simulink model "IEEE34bus_2subsystem"  (R2022b)
settings: Solver=ode4  StartTime=0.0  StopTime=inf  FixedStep=Ts  MaxStep=1e-4  RelTol=1e-4
InitFcn:
  | a=1; % Loading Factor
  | Ts=50e-6;
  | % phase to sequence conversion of RXB matrices
  | c=1*exp(sqrt(-1)*(120*pi/180));
  | T=[1 1 1;1 c*c c;1 c c*c];
  | Tinv=1/3*[1 1 1;1 c c*c;1 c*c c];
  | 
  | % Simulation data for the IEEE 34 Node Test Feeder model
  | mi2km = 1.60934;%  miles to km conversion
  | ft2km = 0.0003048; % feet to km conversion
  | ms2F = 1*1e-6/(2*pi*60);% microsiemens to Farads conversion
  | 
  | %% Configuration 300 - series reactance - ohm/mile
  | R_300 = [1.3368 0.2101 0.2130;0.2101 1.3238 0.2066;0.2130 0.2066 1.3294];
  | X_300 = [1.3343 0.5779 0.5015;0.5779 1.3569 0.4591;0.5015 0.4591 1.3471];
  | % charging susceptance - microsiemens/mile
  | B_300 = [5.3350 -1.5313 -0.9943;-1.5313 5.0979 -0.6212;-0.9943 -0.6212 4.8880];
  | 
  | R_300 = R_300/mi2km;
  | Rseq=Tinv*R_300*T;
  | R1_300=Rseq(2,2);R0_300=Rseq(1,1);
  | 
  | L_300 = (X_300/(2*pi*60))/mi2km;
  | Lseq=Tinv*L_300*T;
  | L1_300=Lseq(2,2);L0_300=Lseq(1,1);
  | 
  | C_300 =(B_300*ms2F)/mi2km;
  | Cseq=Tinv*C_300*T;
  | C1_300=Cseq(2,2);C0_300=Cseq(1,1);
  | 
  | %% Configuration 301 - series reactance - ohm/mile
  | R_301 = [1.9300 0.2327 0.2359;0.2327 1.9157 0.2288;0.2359 0.2288 1.9219];
  | X_301 = [1.4115 0.6442 0.5691;0.6442 1.4281 0.5238;0.5691 0.5238 1.4209];
  | % charging susceptance - microsiemens/mile
  | B_301 = [5.1207 -1.4364 -0.9402;-1.4364 4.9055 -0.5951;-0.9402 -0.5951 4.7154];
  | 
  | R_301 = R_301/mi2km;
  | Rseq=Tinv*R_301*T;
  | R1_301=Rseq(2,2);R0_301=Rseq(1,1);
  | 
  | L_301 = (X_301/(2*pi*60))/mi2km;
  | Lseq=Tinv*L_301*T;
  | L1_301=Lseq(2,2);L0_301=Lseq(1,1);
  | 
  | C_301 =(B_301*ms2F)/mi2km;
  | Cseq=Tinv*C_301*T;
  | C1_301=Cseq(2,2);C0_301=Cseq(1,1);
  | 
  | %% Configuration 302 - series reactance - ohm/mile
  | R_302 = [2.7995 0 0;0 0 0;0 0 0];
  | X_302 = [1.4855 0 0;0 0 0;0 0 0];
  | % charging susceptance - microsiemens/mile
  | B_302 = [4.2251 0 0;0 0 0;0 0 0];
  | 
  | R_302 = R_302/mi2km;
  | Rseq=Tinv*R_302*T;
  | R1_302=Rseq(2,2);R0_302=Rseq(1,1);
  | 
  | L_302 = (X_302/(2*pi*60))/mi2km;
  | Lseq=Tinv*L_302*T;
  | ... (+41 lines)
undefined symbols (not defined in the file): find_system, I, Left, MOV_segment19, MOV_segment9, powergui, Right, type, V, X, xn_g1
libraries: spsSeriesRLCBranchLib x75, spsGroundLib x70, spsThreePhaseVIMeasurementLib x37, spsVoltageMeasurementLib x36, spsThreePhaseSeriesRLCLoadLib x32, spsThreePhasePISectionLineLib x24, spsDCVoltageSourceLib x24, ssn_lib x16, spsSeriesRLCLoadLib x14, spsACCurrentSourceLib x12, spsOnDelayLib x12, spsPiSectionLineLib x8
(part 6 of 8)

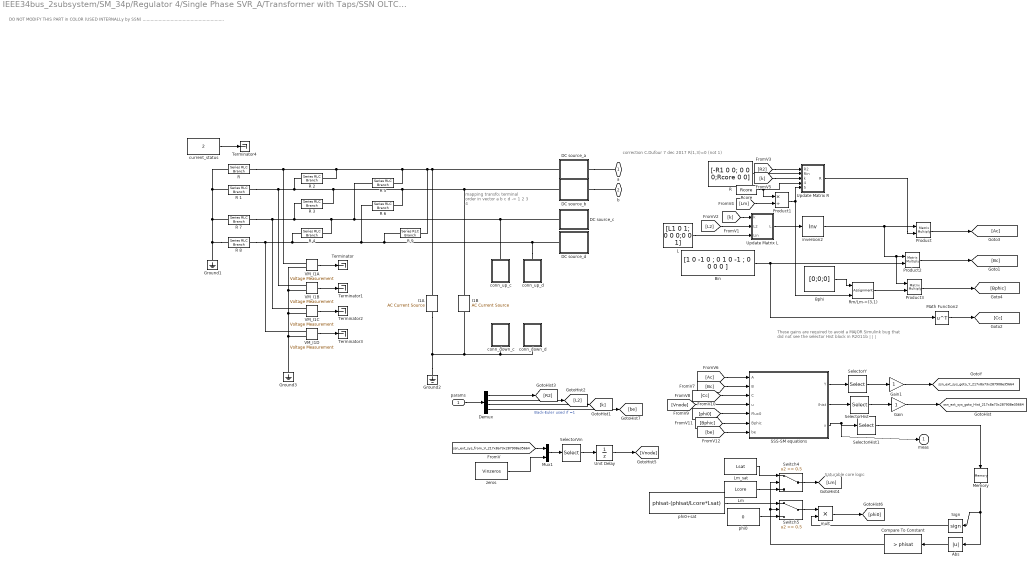
== system IEEE34bus_2subsystem/SM_34p/Regulator 4/Single Phase SVR_A/Transformer with Taps/SSN OLTC xfo v2 ==
  note: correction C.Dufour 7 dec 2017 R(1,3)=0 (not 1)
  note: These gains are required to avoid a MAJOR Simulink bug
      | that did not see the selector Hist block in R2011b
      | |
      | |
      | |
  note: Saturable core logic
  note: DO NOT MODIFY THIS PART in COLOR (USED INTERNALLy by SSN) .............................................................
  note: mapping transfo:
      | terminal    order in vector
      | a b c d -> 1 2 3 4
  params : Inport
  Abs : Abs  SaturateOnIntegerOverflow=off
  Bin : Constant  Value="[1 0 -1  0 ; 0 1 0 -1 ; 0 0 0 0 ]"
  Bphi : Constant  Value=[0;0;0]  VectorParams1D=off
  Compare To Constant : simulink/Logic and Bit Operations/Compare To Constant  relop=>  const=phisat  OutDataTypeStr=uint8
  DC source_a : Subsystem  mask(SSN nodal point interface: DC-source){}
  DC source_b : Subsystem  mask(SSN nodal point interface: DC-source){}
  DC source_c : Subsystem  mask(SSN nodal point interface: DC-source){}
  DC source_d : Subsystem  mask(SSN nodal point interface: DC-source){}
  Demux : Demux
  Gain : Gain
  Gain1 : Gain
  Ground1 : spsGroundLib/Ground  LConnTagsString=a
  Ground2 : spsGroundLib/Ground  LConnTagsString=a
  Ground3 : spsGroundLib/Ground  LConnTagsString=a
  I1A : spsACCurrentSourceLib/AC Current Source  Amplitude=0  Phase=0  Frequency=1928.3746  SampleTime=0  Measurements=None
      settings: LibrarySourceBlock=sps_lib/Sources/AC Current Source
  I1B : spsACCurrentSourceLib/AC Current Source  Amplitude=0  Phase=0  Frequency=1928.3746  SampleTime=0  Measurements=None
      settings: LibrarySourceBlock=sps_lib/Sources/AC Current Source
  L : Constant  Value=[L1 0 1; 0 0 0;0 0 1]
  Lm : Constant  Value=Lcore
  Lm_sat : Constant  Value=Lsat
  Math Function2 : Math  Operator=transpose  SignedPower=on
  Memory : Memory
  Mux1 : Mux  Inputs=2
  Product : Product  Multiplication=Matrix(*)  RndMeth=Zero
  Product1 : Product  Inputs=*/  RndMeth=Zero
  Product2 : Product  Multiplication=Matrix(*)  RndMeth=Zero
  Product3 : Product  Multiplication=Matrix(*)  RndMeth=Zero
  R : Constant  Value=[-R1 0 0; 0 0 0;Rcore 0 0]
  R {,1..9} (10 alike) : spsSeriesRLCBranchLib/Series RLC Branch  LConnTagsString=__new0  RConnTagsString=__new0  BranchType=R  Resistance=1.23456789  Inductance=.5  SetiL0=off  InitialCurrent=0  Capacitance=1.0  Setx0=off  InitialVoltage=0  Measurements=None
  Rcore : Constant  Value=Rcore
  "Rm/Lm->(3,1) " : Assignment  NumberOfDimensions=2  IndexOptions=Index vector (dialog),Index vector (dialog)  Indices=3,1  OutputSizes=1,1
  SSS-SM equations : Subsystem
  SelectorHist : Selector  InputPortWidth=4  IndexOptions=Index vector (dialog)  Indices=hist_sel  OutputSizes=1
  SelectorHist1 : Selector  InputPortWidth=3  IndexOptions=Index vector (dialog)  Indices=3  OutputSizes=1
  SelectorVin : Selector  InputPortWidth=5  IndexOptions=Index vector (dialog)  Indices=vin_sel  OutputSizes=1
  SelectorY : Selector  NumberOfDimensions=2  InputPortWidth=4  IndexOptions=Index vector (dialog),Index vector (dialog)  Indices=hist_sel,hist_sel  OutputSizes=1,1
  Sign : Signum
  Switch4 : Switch  Threshold=0.5  SaturateOnIntegerOverflow=off  InputSameDT=off
  Switch5 : Switch  Threshold=0.5  SaturateOnIntegerOverflow=off  InputSameDT=off
  Terminator{,1..4} (5 alike) : Terminator
  Unit Delay : UnitDelay  SampleTime=Ts  HasFrameUpgradeWarning=on
  Update Matrix L : Subsystem
  Update Matrix R : Subsystem
  VM_I1A : spsVoltageMeasurementLib/Voltage Measurement  PhasorSimulation=off  OutputType=Complex  PSBequivalent=0
  VM_I1B : spsVoltageMeasurementLib/Voltage Measurement  PhasorSimulation=off  OutputType=Complex  PSBequivalent=0
  VM_I1C : spsVoltageMeasurementLib/Voltage Measurement  PhasorSimulation=off  OutputType=Complex  PSBequivalent=0
  VM_I1D : spsVoltageMeasurementLib/Voltage Measurement  PhasorSimulation=off  OutputType=Complex  PSBequivalent=0
  conn_down_c : Subsystem
  conn_down_d : Subsystem
  conn_up_c : Subsystem
  conn_up_d : Subsystem
  current_status : Constant  Value=2
  inversion2 : Product  Inputs=/  Multiplication=Matrix(*)  RndMeth=Zero
  mult : Product
  phi0 : Constant  Value=0
  phi0+sat : Constant  Value=phisat-(phisat/Lcore*Lsat)
  zeros : Constant  Value=Vinzeros
  a : PMIOPort  Side=Left
  b : PMIOPort  Port=2  Side=Right
  meas : Outport  InitialOutput=0  VectorParamsAs1DForOutWhenUnconnected=off
  tag scope: ssn_ext_sys_goto_Hist_217x8a73x287908e35664=global, ssn_ext_sys_goto_Y_217x8a73x287908e35664=global
  wires:
  Gain1/1 -> [ssn_ext_sys_goto_Y_217x8a73x287908e35664]
  Gain/1 -> [ssn_ext_sys_goto_Hist_217x8a73x287908e35664]
  Sign/1 -> mult/2
  mult/1 -> [phi0]
  Switch5/1 -> mult/1
  Unit Delay/1 -> [Vnode]
  params/1 -> Demux/1
  Demux/1 -> [R2]
  Demux/2 -> [L2]
  Demux/3 -> [k]
  Abs/1 -> Compare To Constant/1
  Lm_sat/1 -> Switch4/1
  Lm/1 -> Switch4/3
  Memory/1 -> Abs/1, Sign/1
  phi0/1 -> Switch5/3
  phi0+sat/1 -> Switch5/1
  Switch4/1 -> [Lm]
  Compare To Constant/1 -> Switch4/2, Switch5/2
  [ssn_ext_sys_from_V_217x8a73x287908e35664] -> Mux1/1
  zeros/1 -> Mux1/2
  SelectorVin/1 -> Unit Delay/1
  Mux1/1 -> SelectorVin/1
  current_status/1 -> Terminator4/1
  VM_I1D/1 -> Terminator3/1
  VM_I1C/1 -> Terminator2/1
  VM_I1B/1 -> Terminator1/1
  VM_I1A/1 -> Terminator/1
  L/1 -> Update Matrix L/3(Lin)
  [k] -> Update Matrix L/1(k)
  [L2] -> Update Matrix L/2(L2)
  Update Matrix L/1(L) -> inversion2/1
  R/1 -> Update Matrix R/2(Rin)
  [R2] -> Update Matrix R/1(R2)
  [k] -> Update Matrix R/3(k)
  Rcore/1 -> Update Matrix R/4(Rcore), Product1/1
  inversion2/1 -> Product2/1, Product3/1, Product/1
  [Lm] -> Product1/2
  Product1/1 -> Update Matrix R/5(Rcore/Lcore), "Rm/Lm->(3,1) "/2
  Bin/1 -> Math Function2/1, Product2/2
  Math Function2/1 -> [Cc]
  [Ac] -> SSS-SM equations/1(A)
  [Bc] -> SSS-SM equations/2(B)
  [Cc] -> SSS-SM equations/3(C)
  [Vnode] -> SSS-SM equations/4(u)
  [phi0] -> SSS-SM equations/5(Flux0)
  Bphi/1 -> "Rm/Lm->(3,1) "/1
  [Bphic] -> SSS-SM equations/6(Bphic)
  Product2/1 -> [Bc]
  "Rm/Lm->(3,1) "/1 -> Product3/2
  Update Matrix R/1(R) -> Product/2
  Product/1 -> [Ac]
  Product3/1 -> [Bphic]
  SSS-SM equations/3(x) -> SelectorHist1/1, meas/1
  SelectorHist1/1 -> Memory/1
  [be] -> SSS-SM equations/7(be)
  Demux/4 -> [be]  "Back-Euler used if =1"
  SSS-SM equations/2(Ihist) -> SelectorHist/1
  SSS-SM equations/1(Y) -> SelectorY/1
  SelectorY/1 -> Gain1/1
  SelectorHist/1 -> Gain/1
  connections:
  R 5/RConn1 -- VM_I1A/LConn1 -- "R "/RConn1 -- R 2/RConn1 -- I1A/RConn1 -- DC source_a/LConn1 -- R 9/RConn1
  R 3/RConn1 -- VM_I1B/LConn1 -- R 1/RConn1 -- R 2/LConn1 -- I1B/RConn1 -- DC source_b/LConn1 -- R 6/RConn1
  R 4/RConn1 -- VM_I1C/LConn1 -- R 7/RConn1 -- R 3/LConn1 -- conn_up_c/LConn1 -- DC source_c/LConn1 -- R 5/LConn1
  conn_up_d/LConn1 -- DC source_d/LConn1 -- R 9/LConn1 -- R 6/LConn1 -- VM_I1D/LConn1 -- R 8/RConn1 -- R 4/LConn1
  Ground3/LConn1 -- VM_I1C/LConn2 -- VM_I1A/LConn2 -- VM_I1B/LConn2 -- VM_I1D/LConn2
  DC source_b/RConn1 -- b/RConn1
  Ground2/LConn1 -- I1A/LConn1 -- I1B/LConn1 -- conn_down_c/RConn1 -- conn_down_d/RConn1
  DC source_a/RConn1 -- a/RConn1
  R 8/LConn1 -- Ground1/LConn1 -- R 7/LConn1 -- R 1/LConn1 -- "R "/LConn1

== system IEEE34bus_2subsystem/SM_34p/Regulator 4/Single Phase SVR_A/Voltage Regulator Control/Tap Changer Control ==
  "Up " : Inport
  "Down " : Inport  Port=2
  Constant : Constant  Value=-1
  Constant1 : Constant
  Determine tap position : Subsystem
  Edge Detector : Subsystem  DialogController=POWERSYS.PowerSysDialog  mask(Edge Detector){model=Rising, ic=0}
      mask prompts: model "Edge:"; ic "Input at t = -eps:"
      mask help:
      | This block compares its present input to its previous input.
      |
      | If the input  is a logic signal (TRUE (1) or FALSE (0), the output is a one-step boolean signal TRUE  when  the specified edge (Rising, Falling or Either)  is detected.
      |
      | This block can also be used to detect the slope polarity of a continuous signal. For example, if the specified edge is  "Rising", the output is TRUE as long as the slope of the input signal is positive.
      |
      | The input value at time preceding t=0 is specified by the parameter "Input at t=-eps"
      mask init: same as IEEE34bus_2subsystem/SM_34p/Regulator 3/Single Phase SVR_A/Voltage Regulator Control/Tap Changer Control/Edge Detector
      mask Help: This block is part of a subset of blocks in the Extras library that does not have documentation associated with it, other than the block mask description.
      mask TypeOptions model: Rising | Falling | Either
      mask Display: plot(0,0,100,100, X1,Y1,X2,Y2,X3,Y3,X4,Y4);
  Logical Operator : Logic  Operator=OR  AllPortsSameDT=off
  Logical Operator1 : Logic  AllPortsSameDT=off
  Mechanical Delay : TransportDelay  DelayTime=MecDelay  InitialOutput=InitialPosition  BufferSize=5120
  Memory : Memory  InitialCondition=1  InheritSampleTime=on
  Relational Operator : RelationalOperator  Operator===  OutDataTypeStr=float('double')  InputSameDT=off
  Switch : Switch  Threshold=0.5  InputSameDT=off
  TapNo : Outport  VectorParamsAs1DForOutWhenUnconnected=off
  Ready : Outport  Port=2  VectorParamsAs1DForOutWhenUnconnected=off
  wires:
  Edge Detector/1(Out) -> Logical Operator1/2
  Logical Operator/1 -> Edge Detector/1(In)
  Memory/1 -> Ready/1, Logical Operator1/1
  Relational Operator/1 -> Memory/1
  Determine tap position/1(TapNo) -> Relational Operator/1, Mechanical Delay/1
  Switch/1 -> Determine tap position/1(NewTap)
  Constant1/1 -> Switch/3
  Constant/1 -> Switch/1
  "Down "/1 -> Switch/2, Logical Operator/2
  "Up "/1 -> Logical Operator/1
  Logical Operator1/1 -> Determine tap position/Trigger
  Mechanical Delay/1 -> Relational Operator/2, TapNo/1

== system IEEE34bus_2subsystem/SM_34p/Regulator 4/Single Phase SVR_A/Voltage Regulator Control/Voltage regulator ==
  Vmes (pu) : Inport
  Ready : Inport  Port=2
  RegOn : Inport  Port=3
  Dead Zone : DeadZone  LowerValue=-DeadBand/2  UpperValue=+DeadBand/2
  Discrete Variable Time Delay : spsDiscreteVariableTimeDelayLib/Discrete Variable Time Delay  MaxDelay=3/60+Ts  InitialValue=1  Ts=Ts  DFT=on
      settings: LibrarySourceBlock=|
      | sps_lib/Control/Discrete Variable
      | Time Delay
  Logical Operator : Logic  AllPortsSameDT=off
  Logical Operator1 : Logic  AllPortsSameDT=off
  On Delay : spsOnDelayLib/On Delay  DelayType=On delay  delay=TimeDelay  ic=0  Ts=Ts
  On Delay1 : spsOnDelayLib/On Delay  DelayType=On delay  delay=TimeDelay  ic=0  Ts=Ts
  Relational Operator : RelationalOperator  Operator=>  InputSameDT=off
  Relational Operator1 : RelationalOperator  Operator=<  InputSameDT=off
  Sum : Sum  Inputs=|+-  SaturateOnIntegerOverflow=on
  Switch : Switch  Threshold=1.5  InputSameDT=off
  Vref : Constant  Value=Vref
  Vref1 : Constant  Value=0
  Vref2 : Constant  Value=0
  Vref3 : Constant  Value=0
  Vref4 : Constant  Value=3/60
  Up : Outport  VectorParamsAs1DForOutWhenUnconnected=off
  Down : Outport  Port=2  VectorParamsAs1DForOutWhenUnconnected=off
  wires:
  Vref4/1 -> Discrete Variable Time Delay/2
  Discrete Variable Time Delay/1 -> Logical Operator/2, Logical Operator1/1
  Vref3/1 -> Relational Operator1/2
  On Delay1/1 -> Down/1
  Logical Operator1/1 -> On Delay1/1
  Relational Operator1/1 -> Logical Operator1/2
  On Delay/1 -> Up/1
  Logical Operator/1 -> On Delay/1
  Ready/1 -> Discrete Variable Time Delay/1
  Relational Operator/1 -> Logical Operator/1
  Vref1/1 -> Relational Operator/2
  Dead Zone/1 -> Relational Operator/1, Relational Operator1/1
  Vmes (pu)/1 -> Sum/2
  Vref/1 -> Sum/1
  Sum/1 -> Switch/1
  Switch/1 -> Dead Zone/1
  RegOn/1 -> Switch/2
  Vref2/1 -> Switch/3

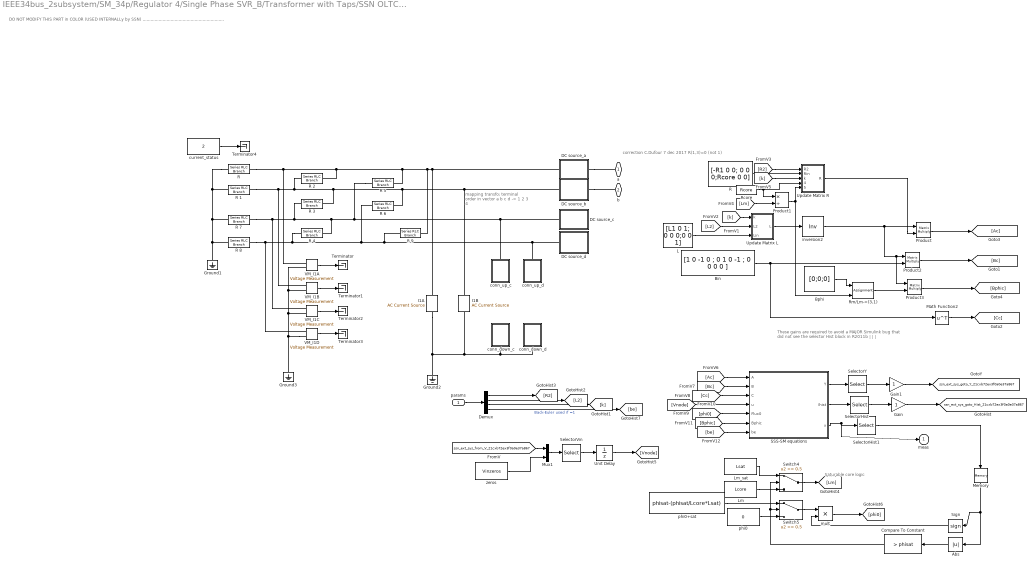
== system IEEE34bus_2subsystem/SM_34p/Regulator 4/Single Phase SVR_B/Transformer with Taps/SSN OLTC xfo v2 ==
  note: mapping transfo:
      | terminal    order in vector
      | a b c d -> 1 2 3 4
  note: DO NOT MODIFY THIS PART in COLOR (USED INTERNALLy by SSN) .............................................................
  note: Saturable core logic
  note: These gains are required to avoid a MAJOR Simulink bug
      | that did not see the selector Hist block in R2011b
      | |
      | |
      | |
  note: correction C.Dufour 7 dec 2017 R(1,3)=0 (not 1)
  params : Inport
  Abs : Abs  SaturateOnIntegerOverflow=off
  Bin : Constant  Value="[1 0 -1  0 ; 0 1 0 -1 ; 0 0 0 0 ]"
  Bphi : Constant  Value=[0;0;0]  VectorParams1D=off
  Compare To Constant : simulink/Logic and Bit Operations/Compare To Constant  relop=>  const=phisat  OutDataTypeStr=uint8
  DC source_a : Subsystem  mask(SSN nodal point interface: DC-source){}
  DC source_b : Subsystem  mask(SSN nodal point interface: DC-source){}
  DC source_c : Subsystem  mask(SSN nodal point interface: DC-source){}
  DC source_d : Subsystem  mask(SSN nodal point interface: DC-source){}
  Demux : Demux
  Gain : Gain
  Gain1 : Gain
  Ground1 : spsGroundLib/Ground  LConnTagsString=a
  Ground2 : spsGroundLib/Ground  LConnTagsString=a
  Ground3 : spsGroundLib/Ground  LConnTagsString=a
  I1A : spsACCurrentSourceLib/AC Current Source  Amplitude=0  Phase=0  Frequency=1928.3746  SampleTime=0  Measurements=None
      settings: LibrarySourceBlock=sps_lib/Sources/AC Current Source
  I1B : spsACCurrentSourceLib/AC Current Source  Amplitude=0  Phase=0  Frequency=1928.3746  SampleTime=0  Measurements=None
      settings: LibrarySourceBlock=sps_lib/Sources/AC Current Source
  L : Constant  Value=[L1 0 1; 0 0 0;0 0 1]
  Lm : Constant  Value=Lcore
  Lm_sat : Constant  Value=Lsat
  Math Function2 : Math  Operator=transpose  SignedPower=on
  Memory : Memory
  Mux1 : Mux  Inputs=2
  Product : Product  Multiplication=Matrix(*)  RndMeth=Zero
  Product1 : Product  Inputs=*/  RndMeth=Zero
  Product2 : Product  Multiplication=Matrix(*)  RndMeth=Zero
  Product3 : Product  Multiplication=Matrix(*)  RndMeth=Zero
  R : Constant  Value=[-R1 0 0; 0 0 0;Rcore 0 0]
  R {,1..9} (10 alike) : spsSeriesRLCBranchLib/Series RLC Branch  LConnTagsString=__new0  RConnTagsString=__new0  BranchType=R  Resistance=1.23456789  Inductance=.5  SetiL0=off  InitialCurrent=0  Capacitance=1.0  Setx0=off  InitialVoltage=0  Measurements=None
  Rcore : Constant  Value=Rcore
  "Rm/Lm->(3,1) " : Assignment  NumberOfDimensions=2  IndexOptions=Index vector (dialog),Index vector (dialog)  Indices=3,1  OutputSizes=1,1
  SSS-SM equations : Subsystem
  SelectorHist : Selector  InputPortWidth=4  IndexOptions=Index vector (dialog)  Indices=hist_sel  OutputSizes=1
  SelectorHist1 : Selector  InputPortWidth=3  IndexOptions=Index vector (dialog)  Indices=3  OutputSizes=1
  SelectorVin : Selector  InputPortWidth=5  IndexOptions=Index vector (dialog)  Indices=vin_sel  OutputSizes=1
  SelectorY : Selector  NumberOfDimensions=2  InputPortWidth=4  IndexOptions=Index vector (dialog),Index vector (dialog)  Indices=hist_sel,hist_sel  OutputSizes=1,1
  Sign : Signum
  Switch4 : Switch  Threshold=0.5  SaturateOnIntegerOverflow=off  InputSameDT=off
  Switch5 : Switch  Threshold=0.5  SaturateOnIntegerOverflow=off  InputSameDT=off
  Terminator{,1..4} (5 alike) : Terminator
  Unit Delay : UnitDelay  SampleTime=Ts  HasFrameUpgradeWarning=on
  Update Matrix L : Subsystem
  Update Matrix R : Subsystem
  VM_I1A : spsVoltageMeasurementLib/Voltage Measurement  PhasorSimulation=off  OutputType=Complex  PSBequivalent=0
  VM_I1B : spsVoltageMeasurementLib/Voltage Measurement  PhasorSimulation=off  OutputType=Complex  PSBequivalent=0
  VM_I1C : spsVoltageMeasurementLib/Voltage Measurement  PhasorSimulation=off  OutputType=Complex  PSBequivalent=0
  VM_I1D : spsVoltageMeasurementLib/Voltage Measurement  PhasorSimulation=off  OutputType=Complex  PSBequivalent=0
  conn_down_c : Subsystem
  conn_down_d : Subsystem
  conn_up_c : Subsystem
  conn_up_d : Subsystem
  current_status : Constant  Value=2
  inversion2 : Product  Inputs=/  Multiplication=Matrix(*)  RndMeth=Zero
  mult : Product
  phi0 : Constant  Value=0
  phi0+sat : Constant  Value=phisat-(phisat/Lcore*Lsat)
  zeros : Constant  Value=Vinzeros
  a : PMIOPort  Side=Left
  b : PMIOPort  Port=2  Side=Right
  meas : Outport  InitialOutput=0  VectorParamsAs1DForOutWhenUnconnected=off
  tag scope: ssn_ext_sys_goto_Hist_21cxb72ex3f0a0e37a867=global, ssn_ext_sys_goto_Y_21cxb72ex3f0a0e37a867=global
  wires:
  SelectorHist/1 -> Gain/1
  SelectorY/1 -> Gain1/1
  SSS-SM equations/1(Y) -> SelectorY/1
  SSS-SM equations/2(Ihist) -> SelectorHist/1
  Demux/4 -> [be]  "Back-Euler used if =1"
  [be] -> SSS-SM equations/7(be)
  SelectorHist1/1 -> Memory/1
  SSS-SM equations/3(x) -> meas/1, SelectorHist1/1
  Product3/1 -> [Bphic]
  Product/1 -> [Ac]
  Update Matrix R/1(R) -> Product/2
  "Rm/Lm->(3,1) "/1 -> Product3/2
  Product2/1 -> [Bc]
  [Bphic] -> SSS-SM equations/6(Bphic)
  Bphi/1 -> "Rm/Lm->(3,1) "/1
  [phi0] -> SSS-SM equations/5(Flux0)
  [Vnode] -> SSS-SM equations/4(u)
  [Cc] -> SSS-SM equations/3(C)
  [Bc] -> SSS-SM equations/2(B)
  [Ac] -> SSS-SM equations/1(A)
  Math Function2/1 -> [Cc]
  Bin/1 -> Product2/2, Math Function2/1
  Product1/1 -> "Rm/Lm->(3,1) "/2, Update Matrix R/5(Rcore/Lcore)
  [Lm] -> Product1/2
  inversion2/1 -> Product/1, Product3/1, Product2/1
  Rcore/1 -> Product1/1, Update Matrix R/4(Rcore)
  [k] -> Update Matrix R/3(k)
  [R2] -> Update Matrix R/1(R2)
  R/1 -> Update Matrix R/2(Rin)
  Update Matrix L/1(L) -> inversion2/1
  [L2] -> Update Matrix L/2(L2)
  [k] -> Update Matrix L/1(k)
  L/1 -> Update Matrix L/3(Lin)
  VM_I1A/1 -> Terminator/1
  VM_I1B/1 -> Terminator1/1
  VM_I1C/1 -> Terminator2/1
  VM_I1D/1 -> Terminator3/1
  current_status/1 -> Terminator4/1
  Mux1/1 -> SelectorVin/1
  SelectorVin/1 -> Unit Delay/1
  zeros/1 -> Mux1/2
  [ssn_ext_sys_from_V_21cxb72ex3f0a0e37a867] -> Mux1/1
  Compare To Constant/1 -> Switch5/2, Switch4/2
  Switch4/1 -> [Lm]
  phi0+sat/1 -> Switch5/1
  phi0/1 -> Switch5/3
  Memory/1 -> Sign/1, Abs/1
  Lm/1 -> Switch4/3
  Lm_sat/1 -> Switch4/1
  Abs/1 -> Compare To Constant/1
  Demux/3 -> [k]
  Demux/2 -> [L2]
  Demux/1 -> [R2]
  params/1 -> Demux/1
  Unit Delay/1 -> [Vnode]
  Switch5/1 -> mult/1
  mult/1 -> [phi0]
  Sign/1 -> mult/2
  Gain/1 -> [ssn_ext_sys_goto_Hist_21cxb72ex3f0a0e37a867]
  Gain1/1 -> [ssn_ext_sys_goto_Y_21cxb72ex3f0a0e37a867]
  connections:
  "R "/LConn1 -- R 1/LConn1 -- R 7/LConn1 -- Ground1/LConn1 -- R 8/LConn1
  DC source_a/RConn1 -- a/RConn1
  conn_down_d/RConn1 -- conn_down_c/RConn1 -- I1B/LConn1 -- I1A/LConn1 -- Ground2/LConn1
  DC source_b/RConn1 -- b/RConn1
  VM_I1D/LConn2 -- VM_I1B/LConn2 -- VM_I1A/LConn2 -- VM_I1C/LConn2 -- Ground3/LConn1
  R 4/LConn1 -- R 8/RConn1 -- VM_I1D/LConn1 -- R 6/LConn1 -- R 9/LConn1 -- DC source_d/LConn1 -- conn_up_d/LConn1
  R 5/LConn1 -- DC source_c/LConn1 -- conn_up_c/LConn1 -- R 3/LConn1 -- R 7/RConn1 -- VM_I1C/LConn1 -- R 4/RConn1
  R 6/RConn1 -- DC source_b/LConn1 -- I1B/RConn1 -- R 2/LConn1 -- R 1/RConn1 -- VM_I1B/LConn1 -- R 3/RConn1
  R 9/RConn1 -- DC source_a/LConn1 -- I1A/RConn1 -- R 2/RConn1 -- "R "/RConn1 -- VM_I1A/LConn1 -- R 5/RConn1

== system IEEE34bus_2subsystem/SM_34p/Regulator 4/Single Phase SVR_B/Voltage Regulator Control/Tap Changer Control ==
  "Up " : Inport
  "Down " : Inport  Port=2
  Constant : Constant  Value=-1
  Constant1 : Constant
  Determine tap position : Subsystem
  Edge Detector : Subsystem  DialogController=POWERSYS.PowerSysDialog  mask(Edge Detector){model=Rising, ic=0}
      mask prompts: model "Edge:"; ic "Input at t = -eps:"
      mask help:
      | This block compares its present input to its previous input.
      |
      | If the input  is a logic signal (TRUE (1) or FALSE (0), the output is a one-step boolean signal TRUE  when  the specified edge (Rising, Falling or Either)  is detected.
      |
      | This block can also be used to detect the slope polarity of a continuous signal. For example, if the specified edge is  "Rising", the output is TRUE as long as the slope of the input signal is positive.
      |
      | The input value at time preceding t=0 is specified by the parameter "Input at t=-eps"
      mask init: same as IEEE34bus_2subsystem/SM_34p/Regulator 3/Single Phase SVR_A/Voltage Regulator Control/Tap Changer Control/Edge Detector
      mask Help: This block is part of a subset of blocks in the Extras library that does not have documentation associated with it, other than the block mask description.
      mask TypeOptions model: Rising | Falling | Either
      mask Display: plot(0,0,100,100, X1,Y1,X2,Y2,X3,Y3,X4,Y4);
  Logical Operator : Logic  Operator=OR  AllPortsSameDT=off
  Logical Operator1 : Logic  AllPortsSameDT=off
  Mechanical Delay : TransportDelay  DelayTime=MecDelay  InitialOutput=InitialPosition  BufferSize=5120
  Memory : Memory  InitialCondition=1  InheritSampleTime=on
  Relational Operator : RelationalOperator  Operator===  OutDataTypeStr=float('double')  InputSameDT=off
  Switch : Switch  Threshold=0.5  InputSameDT=off
  TapNo : Outport  VectorParamsAs1DForOutWhenUnconnected=off
  Ready : Outport  Port=2  VectorParamsAs1DForOutWhenUnconnected=off
  wires:
  Mechanical Delay/1 -> TapNo/1, Relational Operator/2
  Logical Operator1/1 -> Determine tap position/Trigger
  "Up "/1 -> Logical Operator/1
  "Down "/1 -> Logical Operator/2, Switch/2
  Constant/1 -> Switch/1
  Constant1/1 -> Switch/3
  Switch/1 -> Determine tap position/1(NewTap)
  Determine tap position/1(TapNo) -> Mechanical Delay/1, Relational Operator/1
  Relational Operator/1 -> Memory/1
  Memory/1 -> Logical Operator1/1, Ready/1
  Logical Operator/1 -> Edge Detector/1(In)
  Edge Detector/1(Out) -> Logical Operator1/2

== system IEEE34bus_2subsystem/SM_34p/Regulator 4/Single Phase SVR_B/Voltage Regulator Control/Voltage regulator ==
  Vmes (pu) : Inport
  Ready : Inport  Port=2
  RegOn : Inport  Port=3
  Dead Zone : DeadZone  LowerValue=-DeadBand/2  UpperValue=+DeadBand/2
  Discrete Variable Time Delay : spsDiscreteVariableTimeDelayLib/Discrete Variable Time Delay  MaxDelay=3/60+Ts  InitialValue=1  Ts=Ts  DFT=on
      settings: LibrarySourceBlock=|
      | sps_lib/Control/Discrete Variable
      | Time Delay
  Logical Operator : Logic  AllPortsSameDT=off
  Logical Operator1 : Logic  AllPortsSameDT=off
  On Delay : spsOnDelayLib/On Delay  DelayType=On delay  delay=TimeDelay  ic=0  Ts=Ts
  On Delay1 : spsOnDelayLib/On Delay  DelayType=On delay  delay=TimeDelay  ic=0  Ts=Ts
  Relational Operator : RelationalOperator  Operator=>  InputSameDT=off
  Relational Operator1 : RelationalOperator  Operator=<  InputSameDT=off
  Sum : Sum  Inputs=|+-  SaturateOnIntegerOverflow=on
  Switch : Switch  Threshold=1.5  InputSameDT=off
  Vref : Constant  Value=Vref
  Vref1 : Constant  Value=0
  Vref2 : Constant  Value=0
  Vref3 : Constant  Value=0
  Vref4 : Constant  Value=3/60
  Up : Outport  VectorParamsAs1DForOutWhenUnconnected=off
  Down : Outport  Port=2  VectorParamsAs1DForOutWhenUnconnected=off
  wires:
  Vref2/1 -> Switch/3
  RegOn/1 -> Switch/2
  Switch/1 -> Dead Zone/1
  Sum/1 -> Switch/1
  Vref/1 -> Sum/1
  Vmes (pu)/1 -> Sum/2
  Dead Zone/1 -> Relational Operator1/1, Relational Operator/1
  Vref1/1 -> Relational Operator/2
  Relational Operator/1 -> Logical Operator/1
  Ready/1 -> Discrete Variable Time Delay/1
  Logical Operator/1 -> On Delay/1
  On Delay/1 -> Up/1
  Relational Operator1/1 -> Logical Operator1/2
  Logical Operator1/1 -> On Delay1/1
  On Delay1/1 -> Down/1
  Vref3/1 -> Relational Operator1/2
  Discrete Variable Time Delay/1 -> Logical Operator1/1, Logical Operator/2
  Vref4/1 -> Discrete Variable Time Delay/2

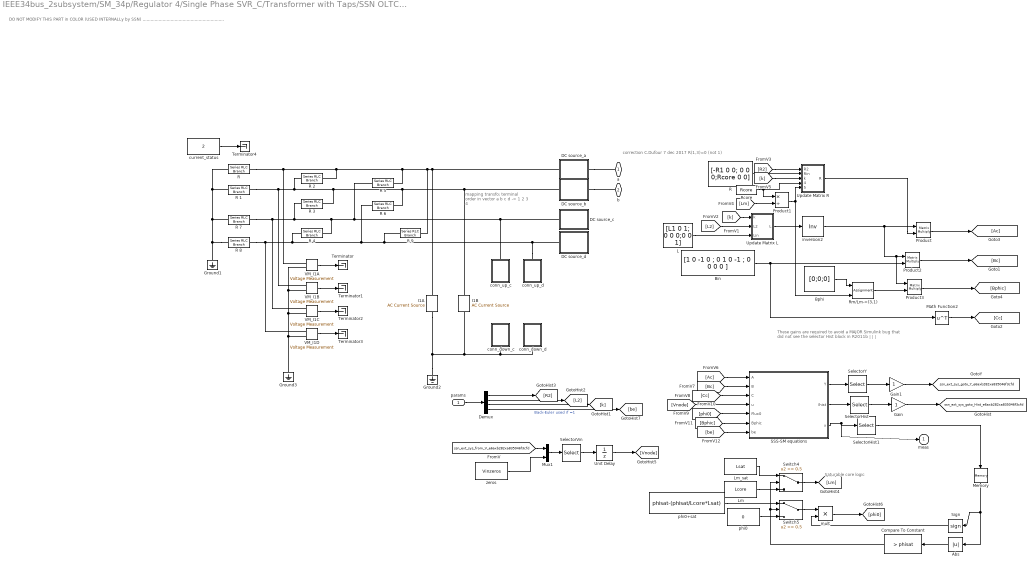
== system IEEE34bus_2subsystem/SM_34p/Regulator 4/Single Phase SVR_C/Transformer with Taps/SSN OLTC xfo v2 ==
  note: correction C.Dufour 7 dec 2017 R(1,3)=0 (not 1)
  note: These gains are required to avoid a MAJOR Simulink bug
      | that did not see the selector Hist block in R2011b
      | |
      | |
      | |
  note: Saturable core logic
  note: DO NOT MODIFY THIS PART in COLOR (USED INTERNALLy by SSN) .............................................................
  note: mapping transfo:
      | terminal    order in vector
      | a b c d -> 1 2 3 4
  params : Inport
  Abs : Abs  SaturateOnIntegerOverflow=off
  Bin : Constant  Value="[1 0 -1  0 ; 0 1 0 -1 ; 0 0 0 0 ]"
  Bphi : Constant  Value=[0;0;0]  VectorParams1D=off
  Compare To Constant : simulink/Logic and Bit Operations/Compare To Constant  relop=>  const=phisat  OutDataTypeStr=uint8
  DC source_a : Subsystem  mask(SSN nodal point interface: DC-source){}
  DC source_b : Subsystem  mask(SSN nodal point interface: DC-source){}
  DC source_c : Subsystem  mask(SSN nodal point interface: DC-source){}
  DC source_d : Subsystem  mask(SSN nodal point interface: DC-source){}
  Demux : Demux
  Gain : Gain
  Gain1 : Gain
  Ground1 : spsGroundLib/Ground  LConnTagsString=a
  Ground2 : spsGroundLib/Ground  LConnTagsString=a
  Ground3 : spsGroundLib/Ground  LConnTagsString=a
  I1A : spsACCurrentSourceLib/AC Current Source  Amplitude=0  Phase=0  Frequency=1928.3746  SampleTime=0  Measurements=None
      settings: LibrarySourceBlock=sps_lib/Sources/AC Current Source
  I1B : spsACCurrentSourceLib/AC Current Source  Amplitude=0  Phase=0  Frequency=1928.3746  SampleTime=0  Measurements=None
      settings: LibrarySourceBlock=sps_lib/Sources/AC Current Source
  L : Constant  Value=[L1 0 1; 0 0 0;0 0 1]
  Lm : Constant  Value=Lcore
  Lm_sat : Constant  Value=Lsat
  Math Function2 : Math  Operator=transpose  SignedPower=on
  Memory : Memory
  Mux1 : Mux  Inputs=2
  Product : Product  Multiplication=Matrix(*)  RndMeth=Zero
  Product1 : Product  Inputs=*/  RndMeth=Zero
  Product2 : Product  Multiplication=Matrix(*)  RndMeth=Zero
  Product3 : Product  Multiplication=Matrix(*)  RndMeth=Zero
  R : Constant  Value=[-R1 0 0; 0 0 0;Rcore 0 0]
  R {,1..9} (10 alike) : spsSeriesRLCBranchLib/Series RLC Branch  LConnTagsString=__new0  RConnTagsString=__new0  BranchType=R  Resistance=1.23456789  Inductance=.5  SetiL0=off  InitialCurrent=0  Capacitance=1.0  Setx0=off  InitialVoltage=0  Measurements=None
  Rcore : Constant  Value=Rcore
  "Rm/Lm->(3,1) " : Assignment  NumberOfDimensions=2  IndexOptions=Index vector (dialog),Index vector (dialog)  Indices=3,1  OutputSizes=1,1
  SSS-SM equations : Subsystem
  SelectorHist : Selector  InputPortWidth=4  IndexOptions=Index vector (dialog)  Indices=hist_sel  OutputSizes=1
  SelectorHist1 : Selector  InputPortWidth=3  IndexOptions=Index vector (dialog)  Indices=3  OutputSizes=1
  SelectorVin : Selector  InputPortWidth=5  IndexOptions=Index vector (dialog)  Indices=vin_sel  OutputSizes=1
  SelectorY : Selector  NumberOfDimensions=2  InputPortWidth=4  IndexOptions=Index vector (dialog),Index vector (dialog)  Indices=hist_sel,hist_sel  OutputSizes=1,1
  Sign : Signum
  Switch4 : Switch  Threshold=0.5  SaturateOnIntegerOverflow=off  InputSameDT=off
  Switch5 : Switch  Threshold=0.5  SaturateOnIntegerOverflow=off  InputSameDT=off
  Terminator{,1..4} (5 alike) : Terminator
  Unit Delay : UnitDelay  SampleTime=Ts  HasFrameUpgradeWarning=on
  Update Matrix L : Subsystem
  Update Matrix R : Subsystem
  VM_I1A : spsVoltageMeasurementLib/Voltage Measurement  PhasorSimulation=off  OutputType=Complex  PSBequivalent=0
  VM_I1B : spsVoltageMeasurementLib/Voltage Measurement  PhasorSimulation=off  OutputType=Complex  PSBequivalent=0
  VM_I1C : spsVoltageMeasurementLib/Voltage Measurement  PhasorSimulation=off  OutputType=Complex  PSBequivalent=0
  VM_I1D : spsVoltageMeasurementLib/Voltage Measurement  PhasorSimulation=off  OutputType=Complex  PSBequivalent=0
  conn_down_c : Subsystem
  conn_down_d : Subsystem
  conn_up_c : Subsystem
  conn_up_d : Subsystem
  current_status : Constant  Value=2
  inversion2 : Product  Inputs=/  Multiplication=Matrix(*)  RndMeth=Zero
  mult : Product
  phi0 : Constant  Value=0
  phi0+sat : Constant  Value=phisat-(phisat/Lcore*Lsat)
  zeros : Constant  Value=Vinzeros
  a : PMIOPort  Side=Left
  b : PMIOPort  Port=2  Side=Right
  meas : Outport  InitialOutput=0  VectorParamsAs1DForOutWhenUnconnected=off
  tag scope: ssn_ext_sys_goto_Hist_e6axb282xa835046f3cfd=global, ssn_ext_sys_goto_Y_e6axb282xa835046f3cfd=global
  wires:
  Gain1/1 -> [ssn_ext_sys_goto_Y_e6axb282xa835046f3cfd]
  Gain/1 -> [ssn_ext_sys_goto_Hist_e6axb282xa835046f3cfd]
  Sign/1 -> mult/2
  mult/1 -> [phi0]
  Switch5/1 -> mult/1
  Unit Delay/1 -> [Vnode]
  params/1 -> Demux/1
  Demux/1 -> [R2]
  Demux/2 -> [L2]
  Demux/3 -> [k]
  Abs/1 -> Compare To Constant/1
  Lm_sat/1 -> Switch4/1
  Lm/1 -> Switch4/3
  Memory/1 -> Abs/1, Sign/1
  phi0/1 -> Switch5/3
  phi0+sat/1 -> Switch5/1
  Switch4/1 -> [Lm]
  Compare To Constant/1 -> Switch4/2, Switch5/2
  [ssn_ext_sys_from_V_e6axb282xa835046f3cfd] -> Mux1/1
  zeros/1 -> Mux1/2
  SelectorVin/1 -> Unit Delay/1
  Mux1/1 -> SelectorVin/1
  current_status/1 -> Terminator4/1
  VM_I1D/1 -> Terminator3/1
  VM_I1C/1 -> Terminator2/1
  VM_I1B/1 -> Terminator1/1
  VM_I1A/1 -> Terminator/1
  L/1 -> Update Matrix L/3(Lin)
  [k] -> Update Matrix L/1(k)
  [L2] -> Update Matrix L/2(L2)
  Update Matrix L/1(L) -> inversion2/1
  R/1 -> Update Matrix R/2(Rin)
  [R2] -> Update Matrix R/1(R2)
  [k] -> Update Matrix R/3(k)
  Rcore/1 -> Update Matrix R/4(Rcore), Product1/1
  inversion2/1 -> Product2/1, Product3/1, Product/1
  [Lm] -> Product1/2
  Product1/1 -> Update Matrix R/5(Rcore/Lcore), "Rm/Lm->(3,1) "/2
  Bin/1 -> Math Function2/1, Product2/2
  Math Function2/1 -> [Cc]
  [Ac] -> SSS-SM equations/1(A)
  [Bc] -> SSS-SM equations/2(B)
  [Cc] -> SSS-SM equations/3(C)
  [Vnode] -> SSS-SM equations/4(u)
  [phi0] -> SSS-SM equations/5(Flux0)
  Bphi/1 -> "Rm/Lm->(3,1) "/1
  [Bphic] -> SSS-SM equations/6(Bphic)
  Product2/1 -> [Bc]
  "Rm/Lm->(3,1) "/1 -> Product3/2
  Update Matrix R/1(R) -> Product/2
  Product/1 -> [Ac]
  Product3/1 -> [Bphic]
  SSS-SM equations/3(x) -> SelectorHist1/1, meas/1
  SelectorHist1/1 -> Memory/1
  [be] -> SSS-SM equations/7(be)
  Demux/4 -> [be]  "Back-Euler used if =1"
  SSS-SM equations/2(Ihist) -> SelectorHist/1
  SSS-SM equations/1(Y) -> SelectorY/1
  SelectorY/1 -> Gain1/1
  SelectorHist/1 -> Gain/1
  connections:
  R 5/RConn1 -- VM_I1A/LConn1 -- "R "/RConn1 -- R 2/RConn1 -- I1A/RConn1 -- DC source_a/LConn1 -- R 9/RConn1
  R 3/RConn1 -- VM_I1B/LConn1 -- R 1/RConn1 -- R 2/LConn1 -- I1B/RConn1 -- DC source_b/LConn1 -- R 6/RConn1
  R 4/RConn1 -- VM_I1C/LConn1 -- R 7/RConn1 -- R 3/LConn1 -- conn_up_c/LConn1 -- DC source_c/LConn1 -- R 5/LConn1
  conn_up_d/LConn1 -- DC source_d/LConn1 -- R 9/LConn1 -- R 6/LConn1 -- VM_I1D/LConn1 -- R 8/RConn1 -- R 4/LConn1
  Ground3/LConn1 -- VM_I1C/LConn2 -- VM_I1A/LConn2 -- VM_I1B/LConn2 -- VM_I1D/LConn2
  DC source_b/RConn1 -- b/RConn1
  Ground2/LConn1 -- I1A/LConn1 -- I1B/LConn1 -- conn_down_c/RConn1 -- conn_down_d/RConn1
  DC source_a/RConn1 -- a/RConn1
  R 8/LConn1 -- Ground1/LConn1 -- R 7/LConn1 -- R 1/LConn1 -- "R "/LConn1

== system IEEE34bus_2subsystem/SM_34p/Regulator 4/Single Phase SVR_C/Voltage Regulator Control/Tap Changer Control ==
  "Up " : Inport
  "Down " : Inport  Port=2
  Constant : Constant  Value=-1
  Constant1 : Constant
  Determine tap position : Subsystem
  Edge Detector : Subsystem  DialogController=POWERSYS.PowerSysDialog  mask(Edge Detector){model=Rising, ic=0}
      mask prompts: model "Edge:"; ic "Input at t = -eps:"
      mask help:
      | This block compares its present input to its previous input.
      |
      | If the input  is a logic signal (TRUE (1) or FALSE (0), the output is a one-step boolean signal TRUE  when  the specified edge (Rising, Falling or Either)  is detected.
      |
      | This block can also be used to detect the slope polarity of a continuous signal. For example, if the specified edge is  "Rising", the output is TRUE as long as the slope of the input signal is positive.
      |
      | The input value at time preceding t=0 is specified by the parameter "Input at t=-eps"
      mask init: same as IEEE34bus_2subsystem/SM_34p/Regulator 3/Single Phase SVR_A/Voltage Regulator Control/Tap Changer Control/Edge Detector
      mask Help: This block is part of a subset of blocks in the Extras library that does not have documentation associated with it, other than the block mask description.
      mask TypeOptions model: Rising | Falling | Either
      mask Display: plot(0,0,100,100, X1,Y1,X2,Y2,X3,Y3,X4,Y4);
  Logical Operator : Logic  Operator=OR  AllPortsSameDT=off
  Logical Operator1 : Logic  AllPortsSameDT=off
  Mechanical Delay : TransportDelay  DelayTime=MecDelay  InitialOutput=InitialPosition  BufferSize=5120
  Memory : Memory  InitialCondition=1  InheritSampleTime=on
  Relational Operator : RelationalOperator  Operator===  OutDataTypeStr=float('double')  InputSameDT=off
  Switch : Switch  Threshold=0.5  InputSameDT=off
  TapNo : Outport  VectorParamsAs1DForOutWhenUnconnected=off
  Ready : Outport  Port=2  VectorParamsAs1DForOutWhenUnconnected=off
  wires:
  Edge Detector/1(Out) -> Logical Operator1/2
  Logical Operator/1 -> Edge Detector/1(In)
  Memory/1 -> Ready/1, Logical Operator1/1
  Relational Operator/1 -> Memory/1
  Determine tap position/1(TapNo) -> Relational Operator/1, Mechanical Delay/1
  Switch/1 -> Determine tap position/1(NewTap)
  Constant1/1 -> Switch/3
  Constant/1 -> Switch/1
  "Down "/1 -> Switch/2, Logical Operator/2
  "Up "/1 -> Logical Operator/1
  Logical Operator1/1 -> Determine tap position/Trigger
  Mechanical Delay/1 -> Relational Operator/2, TapNo/1

== system IEEE34bus_2subsystem/SM_34p/Regulator 4/Single Phase SVR_C/Voltage Regulator Control/Voltage regulator ==
  Vmes (pu) : Inport
  Ready : Inport  Port=2
  RegOn : Inport  Port=3
  Dead Zone : DeadZone  LowerValue=-DeadBand/2  UpperValue=+DeadBand/2
  Discrete Variable Time Delay : spsDiscreteVariableTimeDelayLib/Discrete Variable Time Delay  MaxDelay=3/60+Ts  InitialValue=1  Ts=Ts  DFT=on
      settings: LibrarySourceBlock=|
      | sps_lib/Control/Discrete Variable
      | Time Delay
  Logical Operator : Logic  AllPortsSameDT=off
  Logical Operator1 : Logic  AllPortsSameDT=off
  On Delay : spsOnDelayLib/On Delay  DelayType=On delay  delay=TimeDelay  ic=0  Ts=Ts
  On Delay1 : spsOnDelayLib/On Delay  DelayType=On delay  delay=TimeDelay  ic=0  Ts=Ts
  Relational Operator : RelationalOperator  Operator=>  InputSameDT=off
  Relational Operator1 : RelationalOperator  Operator=<  InputSameDT=off
  Sum : Sum  Inputs=|+-  SaturateOnIntegerOverflow=on
  Switch : Switch  Threshold=1.5  InputSameDT=off
  Vref : Constant  Value=Vref
  Vref1 : Constant  Value=0
  Vref2 : Constant  Value=0
  Vref3 : Constant  Value=0
  Vref4 : Constant  Value=3/60
  Up : Outport  VectorParamsAs1DForOutWhenUnconnected=off
  Down : Outport  Port=2  VectorParamsAs1DForOutWhenUnconnected=off
  wires:
  Vref4/1 -> Discrete Variable Time Delay/2
  Discrete Variable Time Delay/1 -> Logical Operator/2, Logical Operator1/1
  Vref3/1 -> Relational Operator1/2
  On Delay1/1 -> Down/1
  Logical Operator1/1 -> On Delay1/1
  Relational Operator1/1 -> Logical Operator1/2
  On Delay/1 -> Up/1
  Logical Operator/1 -> On Delay/1
  Ready/1 -> Discrete Variable Time Delay/1
  Relational Operator/1 -> Logical Operator/1
  Vref1/1 -> Relational Operator/2
  Dead Zone/1 -> Relational Operator/1, Relational Operator1/1
  Vmes (pu)/1 -> Sum/2
  Vref/1 -> Sum/1
  Sum/1 -> Switch/1
  Switch/1 -> Dead Zone/1
  RegOn/1 -> Switch/2
  Vref2/1 -> Switch/3

== system IEEE34bus_2subsystem/SM_34p/Regulator 3/Single Phase SVR_A/Transformer with Taps/SSN OLTC xfo v2/DC source_a ==
  I1A_V : spsDCVoltageSourceLib/DC Voltage Source  Amplitude=0  Measurements=None
  Conn1 : PMIOPort  Side=Left
  Conn2 : PMIOPort  Port=2  Side=Right
  connections:
  Conn2/RConn1 -- I1A_V/RConn1
  Conn1/RConn1 -- I1A_V/LConn1

== system IEEE34bus_2subsystem/SM_34p/Regulator 3/Single Phase SVR_A/Transformer with Taps/SSN OLTC xfo v2/DC source_b ==
  I1B_V : spsDCVoltageSourceLib/DC Voltage Source  Amplitude=0  Measurements=None
  Conn3 : PMIOPort  Side=Left
  Conn4 : PMIOPort  Port=2  Side=Right
  connections:
  Conn3/RConn1 -- I1B_V/LConn1
  Conn4/RConn1 -- I1B_V/RConn1

== system IEEE34bus_2subsystem/SM_34p/Regulator 3/Single Phase SVR_A/Transformer with Taps/SSN OLTC xfo v2/DC source_c ==
  I1C_V : spsDCVoltageSourceLib/DC Voltage Source  Amplitude=0  Measurements=None
  Conn1 : PMIOPort  Side=Left
  Conn2 : PMIOPort  Port=2  Side=Right
  connections:
  Conn1/RConn1 -- I1C_V/LConn1
  Conn2/RConn1 -- I1C_V/RConn1

== system IEEE34bus_2subsystem/SM_34p/Regulator 3/Single Phase SVR_A/Transformer with Taps/SSN OLTC xfo v2/DC source_d ==
  I1D_V : spsDCVoltageSourceLib/DC Voltage Source  Amplitude=0  Measurements=None
  Conn3 : PMIOPort  Side=Left
  Conn4 : PMIOPort  Port=2  Side=Right
  connections:
  Conn4/RConn1 -- I1D_V/RConn1
  Conn3/RConn1 -- I1D_V/LConn1

== system IEEE34bus_2subsystem/SM_34p/Regulator 3/Single Phase SVR_A/Transformer with Taps/SSN OLTC xfo v2/SSS-SM equations ==
  A : Inport
  B : Inport  Port=2
  C : Inport  Port=3
  u : Inport  Port=4
  Flux0 : Inport  Port=5
  Bphic : Inport  Port=6
  be : Inport  Port=7
  Constant : Constant
  Discretize : Subsystem
  Product{1..3,5..6} (5 alike) : Product  Multiplication=Matrix(*)  SaturateOnIntegerOverflow=on  OutDataTypeStr=Inherit: Same as first input
  Sum1 : Sum  Inputs=-+  SaturateOnIntegerOverflow=on
  Sum2 : Sum  Inputs=+++  SaturateOnIntegerOverflow=on
  Sum3 : Sum  SaturateOnIntegerOverflow=on
  mult1 : Product
  u5 : Constant  Value=eye(3,3)
  z-1 : UnitDelay  SampleTime=Ts  HasFrameUpgradeWarning=on
  Y : Outport  VectorParamsAs1DForOutWhenUnconnected=off
  Ihist : Outport  Port=2  VectorParamsAs1DForOutWhenUnconnected=off
  x : Outport  Port=3  VectorParamsAs1DForOutWhenUnconnected=off
  wires:
  be/1 -> Sum1/1, Discretize/5(be)
  Sum1/1 -> mult1/2  "=1 if trapeze           =0 if BE"
  mult1/1 -> Sum2/2
  Constant/1 -> Sum1/2
  Bphic/1 -> Discretize/4(Bphic)
  Flux0/1 -> Product1/2
  Product1/1 -> Sum2/3
  Discretize/3(Bdin) -> Product1/1
  Discretize/2(Bd) -> Product2/2, Product5/1
  z-1/1 -> Sum3/1
  u/1 -> Product5/2
  Discretize/1(Ad) -> Product3/1
  Sum2/1 -> Product6/2, z-1/1
  Sum3/1 -> x/1, Product3/2  "new_x"
  Product3/1 -> Sum2/1
  Product5/1 -> mult1/1, Sum3/2
  Product6/1 -> Ihist/1
  C/1 -> Product6/1, Product2/1
  B/1 -> Discretize/2(Bc)
  A/1 -> Discretize/1(Ac)
  Product2/1 -> Y/1
  u5/1 -> Discretize/3(Unity)

== system IEEE34bus_2subsystem/SM_34p/Regulator 3/Single Phase SVR_A/Transformer with Taps/SSN OLTC xfo v2/Update Matrix L ==
  k : Inport
  L2 : Inport  Port=2
  Lin : Inport  Port=3
  "L2->(2,2) " : Assignment  NumberOfDimensions=2  IndexOptions=Index vector (dialog),Index vector (dialog)  Indices=[2],[2]  OutputSizes=1,1
  k->(2,3) : Assignment  NumberOfDimensions=2  IndexOptions=Index vector (dialog),Index vector (dialog)  Indices=[2],[3]  OutputSizes=1,1
  L : Outport  VectorParamsAs1DForOutWhenUnconnected=off
  wires:
  k->(2,3)/1 -> "L2->(2,2) "/1
  k/1 -> k->(2,3)/2
  Lin/1 -> k->(2,3)/1
  L2/1 -> "L2->(2,2) "/2
  "L2->(2,2) "/1 -> L/1

== system IEEE34bus_2subsystem/SM_34p/Regulator 3/Single Phase SVR_A/Transformer with Taps/SSN OLTC xfo v2/Update Matrix R ==
  R2 : Inport
  Rin : Inport  Port=2
  k : Inport  Port=3
  Rcore : Inport  Port=4
  Rcore/Lcore : Inport  Port=5
  "-R2->(2,2) " : Assignment  NumberOfDimensions=2  IndexOptions=Index vector (dialog),Index vector (dialog)  Indices=[2],[2]  OutputSizes=1,1
  -Rm/Lm->(3,3) : Assignment  NumberOfDimensions=2  IndexOptions=Index vector (dialog),Index vector (dialog)  Indices=3,3  OutputSizes=1,1
  Gain : Gain  Gain=-1
  Gain1 : Gain  Gain=-1
  Product1 : Product  RndMeth=Zero
  kRm->(3,2) : Assignment  NumberOfDimensions=2  IndexOptions=Index vector (dialog),Index vector (dialog)  Indices=3,2  OutputSizes=1,1
  R : Outport  VectorParamsAs1DForOutWhenUnconnected=off
  wires:
  Rcore/Lcore/1 -> Gain1/1
  Gain1/1 -> -Rm/Lm->(3,3)/2
  Rcore/1 -> Product1/1
  -Rm/Lm->(3,3)/1 -> R/1
  kRm->(3,2)/1 -> -Rm/Lm->(3,3)/1
  Product1/1 -> kRm->(3,2)/2
  k/1 -> Product1/2
  Gain/1 -> "-R2->(2,2) "/2
  Rin/1 -> "-R2->(2,2) "/1
  R2/1 -> Gain/1
  "-R2->(2,2) "/1 -> kRm->(3,2)/1

== system IEEE34bus_2subsystem/SM_34p/Regulator 3/Single Phase SVR_A/Transformer with Taps/SSN OLTC xfo v2/conn_down_c ==
  b2 : PMIOPort  Side=Right
  b1 : PMIOPort  Port=2  Side=Left
  connections:
  b1/RConn1 -- b2/RConn1

== system IEEE34bus_2subsystem/SM_34p/Regulator 3/Single Phase SVR_A/Transformer with Taps/SSN OLTC xfo v2/conn_down_d ==
  b2 : PMIOPort  Side=Right
  b1 : PMIOPort  Port=2  Side=Left
  connections:
  b1/RConn1 -- b2/RConn1

== system IEEE34bus_2subsystem/SM_34p/Regulator 3/Single Phase SVR_A/Transformer with Taps/SSN OLTC xfo v2/conn_up_c ==
  b2 : PMIOPort  Side=Right
  b1 : PMIOPort  Port=2  Side=Left
  connections:
  b1/RConn1 -- b2/RConn1

== system IEEE34bus_2subsystem/SM_34p/Regulator 3/Single Phase SVR_A/Transformer with Taps/SSN OLTC xfo v2/conn_up_d ==
  b2 : PMIOPort  Side=Right
  b1 : PMIOPort  Port=2  Side=Left
  connections:
  b1/RConn1 -- b2/RConn1

== system IEEE34bus_2subsystem/SM_34p/Regulator 3/Single Phase SVR_A/Voltage Regulator Control/Tap Changer Control/Determine tap position ==
  NewTap : Inport
  Trigger : TriggerPort  VariantControl=Variant
  Memory : Memory  InitialCondition=InitialPosition  InheritSampleTime=on
  Saturation : Saturate  UpperLimit=MinMaxTap(2)  LowerLimit=MinMaxTap(1)
  Sum : Sum  Inputs=|++  SaturateOnIntegerOverflow=on
  TapNo : Outport  InitialOutput=InitialPosition  VectorParamsAs1DForOutWhenUnconnected=off
  wires:
  NewTap/1 -> Sum/1
  Sum/1 -> Saturation/1
  Memory/1 -> Sum/2
  Saturation/1 -> TapNo/1, Memory/1

== system IEEE34bus_2subsystem/SM_34p/Regulator 3/Single Phase SVR_A/Voltage Regulator Control/Tap Changer Control/Edge Detector ==
  note: Edge or Slope Detector
  In : Inport
  Constant1 : Constant  Value=model
  Demux : Demux  Outputs=2
      settings: DisplayOption=none
  Logical Operator1 : Logic  Operator=OR
  Memory : Memory  InitialCondition=ic  LinearizeAsDelay=on
  Multiport Switch : MultiPortSwitch  InputSameDT=off
  NEGATIVE Edge : Subsystem  TreatAsAtomicUnit=on
  POSITIVE Edge : Subsystem  TreatAsAtomicUnit=on
  either edge : Constant  Value=[1 1]
  neg. edge : Constant  Value=[0 1]
  pos. edge : Constant  Value=[1 0]
  Out : Outport  VectorParamsAs1DForOutWhenUnconnected=off
  wires:
  either edge/1 -> Multiport Switch/4
  Demux/2 -> NEGATIVE Edge/Enable
  Demux/1 -> POSITIVE Edge/Enable
  Multiport Switch/1 -> Demux/1
  Constant1/1 -> Multiport Switch/1
  neg. edge/1 -> Multiport Switch/3
  pos. edge/1 -> Multiport Switch/2
  In/1 -> Memory/1, NEGATIVE Edge/1(IN), POSITIVE Edge/1(IN)
  Memory/1 -> NEGATIVE Edge/2(IN previous), POSITIVE Edge/2(IN previous)
  POSITIVE Edge/1(OUT) -> Logical Operator1/1
  NEGATIVE Edge/1(OUT) -> Logical Operator1/2
  Logical Operator1/1 -> Out/1

== system IEEE34bus_2subsystem/SM_34p/Regulator 3/Single Phase SVR_B/Transformer with Taps/SSN OLTC xfo v2/DC source_a ==
  I1A_V : spsDCVoltageSourceLib/DC Voltage Source  Amplitude=0  Measurements=None
  Conn1 : PMIOPort  Side=Left
  Conn2 : PMIOPort  Port=2  Side=Right
  connections:
  Conn1/RConn1 -- I1A_V/LConn1
  Conn2/RConn1 -- I1A_V/RConn1

== system IEEE34bus_2subsystem/SM_34p/Regulator 3/Single Phase SVR_B/Transformer with Taps/SSN OLTC xfo v2/DC source_b ==
  I1B_V : spsDCVoltageSourceLib/DC Voltage Source  Amplitude=0  Measurements=None
  Conn3 : PMIOPort  Side=Left
  Conn4 : PMIOPort  Port=2  Side=Right
  connections:
  Conn4/RConn1 -- I1B_V/RConn1
  Conn3/RConn1 -- I1B_V/LConn1

== system IEEE34bus_2subsystem/SM_34p/Regulator 3/Single Phase SVR_B/Transformer with Taps/SSN OLTC xfo v2/DC source_c ==
  I1C_V : spsDCVoltageSourceLib/DC Voltage Source  Amplitude=0  Measurements=None
  Conn1 : PMIOPort  Side=Left
  Conn2 : PMIOPort  Port=2  Side=Right
  connections:
  Conn2/RConn1 -- I1C_V/RConn1
  Conn1/RConn1 -- I1C_V/LConn1

== system IEEE34bus_2subsystem/SM_34p/Regulator 3/Single Phase SVR_B/Transformer with Taps/SSN OLTC xfo v2/DC source_d ==
  I1D_V : spsDCVoltageSourceLib/DC Voltage Source  Amplitude=0  Measurements=None
  Conn3 : PMIOPort  Side=Left
  Conn4 : PMIOPort  Port=2  Side=Right
  connections:
  Conn3/RConn1 -- I1D_V/LConn1
  Conn4/RConn1 -- I1D_V/RConn1

== system IEEE34bus_2subsystem/SM_34p/Regulator 3/Single Phase SVR_B/Transformer with Taps/SSN OLTC xfo v2/SSS-SM equations ==
  A : Inport
  B : Inport  Port=2
  C : Inport  Port=3
  u : Inport  Port=4
  Flux0 : Inport  Port=5
  Bphic : Inport  Port=6
  be : Inport  Port=7
  Constant : Constant
  Discretize : Subsystem
  Product{1..3,5..6} (5 alike) : Product  Multiplication=Matrix(*)  SaturateOnIntegerOverflow=on  OutDataTypeStr=Inherit: Same as first input
  Sum1 : Sum  Inputs=-+  SaturateOnIntegerOverflow=on
  Sum2 : Sum  Inputs=+++  SaturateOnIntegerOverflow=on
  Sum3 : Sum  SaturateOnIntegerOverflow=on
  mult1 : Product
  u5 : Constant  Value=eye(3,3)
  z-1 : UnitDelay  SampleTime=Ts  HasFrameUpgradeWarning=on
  Y : Outport  VectorParamsAs1DForOutWhenUnconnected=off
  Ihist : Outport  Port=2  VectorParamsAs1DForOutWhenUnconnected=off
  x : Outport  Port=3  VectorParamsAs1DForOutWhenUnconnected=off
  wires:
  u5/1 -> Discretize/3(Unity)
  Product2/1 -> Y/1
  A/1 -> Discretize/1(Ac)
  B/1 -> Discretize/2(Bc)
  C/1 -> Product2/1, Product6/1
  Product6/1 -> Ihist/1
  Product5/1 -> Sum3/2, mult1/1
  Product3/1 -> Sum2/1
  Sum3/1 -> Product3/2, x/1  "new_x"
  Sum2/1 -> z-1/1, Product6/2
  Discretize/1(Ad) -> Product3/1
  u/1 -> Product5/2
  z-1/1 -> Sum3/1
  Discretize/2(Bd) -> Product5/1, Product2/2
  Discretize/3(Bdin) -> Product1/1
  Product1/1 -> Sum2/3
  Flux0/1 -> Product1/2
  Bphic/1 -> Discretize/4(Bphic)
  Constant/1 -> Sum1/2
  mult1/1 -> Sum2/2
  Sum1/1 -> mult1/2  "=1 if trapeze           =0 if BE"
  be/1 -> Discretize/5(be), Sum1/1

== system IEEE34bus_2subsystem/SM_34p/Regulator 3/Single Phase SVR_B/Transformer with Taps/SSN OLTC xfo v2/Update Matrix L ==
  k : Inport
  L2 : Inport  Port=2
  Lin : Inport  Port=3
  "L2->(2,2) " : Assignment  NumberOfDimensions=2  IndexOptions=Index vector (dialog),Index vector (dialog)  Indices=[2],[2]  OutputSizes=1,1
  k->(2,3) : Assignment  NumberOfDimensions=2  IndexOptions=Index vector (dialog),Index vector (dialog)  Indices=[2],[3]  OutputSizes=1,1
  L : Outport  VectorParamsAs1DForOutWhenUnconnected=off
  wires:
  "L2->(2,2) "/1 -> L/1
  L2/1 -> "L2->(2,2) "/2
  Lin/1 -> k->(2,3)/1
  k/1 -> k->(2,3)/2
  k->(2,3)/1 -> "L2->(2,2) "/1

== system IEEE34bus_2subsystem/SM_34p/Regulator 3/Single Phase SVR_B/Transformer with Taps/SSN OLTC xfo v2/Update Matrix R ==
  R2 : Inport
  Rin : Inport  Port=2
  k : Inport  Port=3
  Rcore : Inport  Port=4
  Rcore/Lcore : Inport  Port=5
  "-R2->(2,2) " : Assignment  NumberOfDimensions=2  IndexOptions=Index vector (dialog),Index vector (dialog)  Indices=[2],[2]  OutputSizes=1,1
  -Rm/Lm->(3,3) : Assignment  NumberOfDimensions=2  IndexOptions=Index vector (dialog),Index vector (dialog)  Indices=3,3  OutputSizes=1,1
  Gain : Gain  Gain=-1
  Gain1 : Gain  Gain=-1
  Product1 : Product  RndMeth=Zero
  kRm->(3,2) : Assignment  NumberOfDimensions=2  IndexOptions=Index vector (dialog),Index vector (dialog)  Indices=3,2  OutputSizes=1,1
  R : Outport  VectorParamsAs1DForOutWhenUnconnected=off
  wires:
  "-R2->(2,2) "/1 -> kRm->(3,2)/1
  R2/1 -> Gain/1
  Rin/1 -> "-R2->(2,2) "/1
  Gain/1 -> "-R2->(2,2) "/2
  k/1 -> Product1/2
  Product1/1 -> kRm->(3,2)/2
  kRm->(3,2)/1 -> -Rm/Lm->(3,3)/1
  -Rm/Lm->(3,3)/1 -> R/1
  Rcore/1 -> Product1/1
  Gain1/1 -> -Rm/Lm->(3,3)/2
  Rcore/Lcore/1 -> Gain1/1
